simulink model "ISO_PID"  (R2018a)
settings: Solver=FixedStepAuto  StartTime=0.0  StopTime=3000  FixedStep=0.1  RelTol=1e-3
values from neighbouring files (symbols this model uses):
  f = [0,0]    [Model.m]
  h_T = [0 0]    [Model.m]
  hc = minreal(hc)    [Model.m]
libraries: simulink x2
settings Model: Creator=MinhKhanhPC  LastModifiedBy=thanhdo

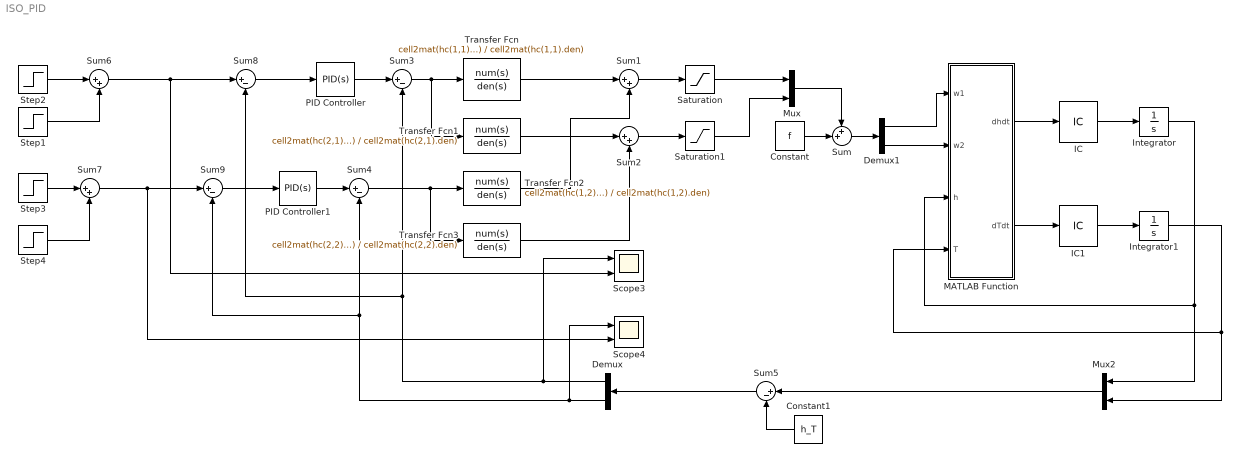
== system ISO_PID ==
  Constant : Constant  Value=f
  Constant1 : Constant  Value=h_T
  Demux : Demux  Outputs=2
  Demux1 : Demux  Outputs=2
  IC : InitialCondition  Value=0.1
  IC1 : InitialCondition  Value=30
  Integrator : Integrator  InitialCondition=0.1
  Integrator1 : Integrator  InitialCondition=30
  MATLAB Function : MATLAB Function  TreatAsAtomicUnit=on
  Mux : Mux  Inputs=2
  Mux2 : Mux  Inputs=2
  PID Controller : simulink/Continuous/PID Controller  Controller=PID  TimeDomain=Continuous-time  SampleTime=-1  IntegratorMethod=Forward Euler  FilterMethod=Forward Euler  Form=Parallel  UseFilter=on  ControllerParametersSource=internal  P=50  I=0.02  D=0  N=100  InitialConditionSource=internal  InitialConditionForIntegrator=0  InitialConditionForFilter=0  ExternalReset=none  LimitOutput=off  UpperSaturationLimit=inf  LowerSaturationLimit=-inf  LinearizeAsGain=on  AntiWindupMode=none  Kb=1  TrackingMode=off  Kt=1  PParamMin=[]  PParamMax=[]  IParamMin=[]  IParamMax=[]  DParamMin=[]  DParamMax=[]  NParamMin=[]  NParamMax=[]  KbParamMin=[]  KbParamMax=[]  KtParamMin=[]  KtParamMax=[]  POutMin=[]  POutMax=[]  IOutMin=[]  IOutMax=[]  DOutMin=[]  DOutMax=[]  NOutMin=[]  NOutMax=[]  KbOutMin=[]  KbOutMax=[]  KtOutMin=[]  KtOutMax=[]  IntegratorOutMin=[]  IntegratorOutMax=[]  FilterOutMin=[]  FilterOutMax=[]  SumOutMin=[]  SumOutMax=[]  SumI1OutMin=[]  SumI1OutMax=[]  SumI2OutMin=[]  SumI2OutMax=[]  SumI3OutMin=[]  SumI3OutMax=[]  SumDOutMin=[]  SumDOutMax=[]  SaturationOutMin=[]  SaturationOutMax=[]  IntegratorContinuousStateAttributes=''  IntegratorStateMustResolveToSignalObject=off  IntegratorRTWStateStorageClass=Auto  FilterContinuousStateAttributes=''  FilterStateMustResolveToSignalObject=off  FilterRTWStateStorageClass=Auto  DifferentiatorICPrevScaledInput=0  DifferentiatorOutMin=[]  DifferentiatorOutMax=[]  FilterDiffOutCoefMin=[]  FilterDiffOutCoefMax=[]  SumDenOutMin=[]  SumDenOutMax=[]  SumNumOutMin=[]  SumNumOutMax=[]  ReciprocalOutMin=[]  ReciprocalOutMax=[]  DivideOutMin=[]  DivideOutMax=[]  TunerSelectOption=Transfer Function Based (PID Tuner App)
  PID Controller1 : simulink/Continuous/PID Controller  Controller=PID  TimeDomain=Continuous-time  SampleTime=-1  IntegratorMethod=Forward Euler  FilterMethod=Forward Euler  Form=Parallel  UseFilter=on  ControllerParametersSource=internal  P=30  I=0  D=0  N=100  InitialConditionSource=internal  InitialConditionForIntegrator=0  InitialConditionForFilter=0  ExternalReset=none  LimitOutput=off  UpperSaturationLimit=inf  LowerSaturationLimit=-inf  LinearizeAsGain=on  AntiWindupMode=none  Kb=1  TrackingMode=off  Kt=1  PParamMin=[]  PParamMax=[]  IParamMin=[]  IParamMax=[]  DParamMin=[]  DParamMax=[]  NParamMin=[]  NParamMax=[]  KbParamMin=[]  KbParamMax=[]  KtParamMin=[]  KtParamMax=[]  POutMin=[]  POutMax=[]  IOutMin=[]  IOutMax=[]  DOutMin=[]  DOutMax=[]  NOutMin=[]  NOutMax=[]  KbOutMin=[]  KbOutMax=[]  KtOutMin=[]  KtOutMax=[]  IntegratorOutMin=[]  IntegratorOutMax=[]  FilterOutMin=[]  FilterOutMax=[]  SumOutMin=[]  SumOutMax=[]  SumI1OutMin=[]  SumI1OutMax=[]  SumI2OutMin=[]  SumI2OutMax=[]  SumI3OutMin=[]  SumI3OutMax=[]  SumDOutMin=[]  SumDOutMax=[]  SaturationOutMin=[]  SaturationOutMax=[]  IntegratorContinuousStateAttributes=''  IntegratorStateMustResolveToSignalObject=off  IntegratorRTWStateStorageClass=Auto  FilterContinuousStateAttributes=''  FilterStateMustResolveToSignalObject=off  FilterRTWStateStorageClass=Auto  DifferentiatorICPrevScaledInput=0  DifferentiatorOutMin=[]  DifferentiatorOutMax=[]  FilterDiffOutCoefMin=[]  FilterDiffOutCoefMax=[]  SumDenOutMin=[]  SumDenOutMax=[]  SumNumOutMin=[]  SumNumOutMax=[]  ReciprocalOutMin=[]  ReciprocalOutMax=[]  DivideOutMin=[]  DivideOutMax=[]  TunerSelectOption=Transfer Function Based (PID Tuner App)
  Saturation : Saturate  UpperLimit=4.28e-5  LowerLimit=0
  Saturation1 : Saturate  UpperLimit=2.28e-5  LowerLimit=0
  Scope3 : Scope  NumInputPorts=2
  Scope4 : Scope  NumInputPorts=2
  Step1 : Step  Time=1000  After=0.05  SampleTime=0
  Step2 : Step  After=0.05  SampleTime=0
  Step3 : Step  After=-5  SampleTime=0
  Step4 : Step  Time=2000  After=3  SampleTime=0
  Sum : Sum  Inputs=++|
  Sum{1..2,6..7} (4 alike) : Sum  Inputs=|++
  Sum{3..5,8..9} (5 alike) : Sum  Inputs=|+-
  Transfer Fcn : TransferFcn  Numerator=cell2mat(hc(1,1).num)  Denominator=cell2mat(hc(1,1).den)
  Transfer Fcn1 : TransferFcn  Numerator=cell2mat(hc(2,1).num)  Denominator=cell2mat(hc(2,1).den)
  Transfer Fcn2 : TransferFcn  Numerator=cell2mat(hc(1,2).num)  Denominator=cell2mat(hc(1,2).den)
  Transfer Fcn3 : TransferFcn  Numerator=cell2mat(hc(2,2).num)  Denominator=cell2mat(hc(2,2).den)
  wires:
  MATLAB Function/1(dhdt) -> IC/1
  Integrator/1 -> Mux2/1, MATLAB Function/3(h)
  Transfer Fcn3/1 -> Sum2/2
  Demux/2 -> Sum9/2, Sum4/2, Scope4/1
  Sum3/1 -> Transfer Fcn1/1, Transfer Fcn/1
  Demux/1 -> Sum8/2, Sum3/2, Scope3/1
  Transfer Fcn1/1 -> Sum2/1
  Transfer Fcn/1 -> Sum1/1
  Transfer Fcn2/1 -> Sum1/2
  Sum4/1 -> Transfer Fcn3/1, Transfer Fcn2/1
  Saturation/1 -> Mux/1
  Saturation1/1 -> Mux/2
  Sum5/1 -> Demux/1
  Constant1/1 -> Sum5/2
  Sum1/1 -> Saturation/1
  Sum2/1 -> Saturation1/1
  Sum/1 -> Demux1/1
  Demux1/1 -> MATLAB Function/1(w1)
  Demux1/2 -> MATLAB Function/2(w2)
  MATLAB Function/2(dTdt) -> IC1/1
  Integrator1/1 -> MATLAB Function/4(T), Mux2/2
  Mux2/1 -> Sum5/1
  IC/1 -> Integrator/1
  IC1/1 -> Integrator1/1
  Step2/1 -> Sum6/1
  Step1/1 -> Sum6/2
  Step3/1 -> Sum7/1
  Step4/1 -> Sum7/2
  PID Controller1/1 -> Sum4/1
  PID Controller/1 -> Sum3/1
  Sum8/1 -> PID Controller/1
  Sum9/1 -> PID Controller1/1
  Constant/1 -> Sum/2
  Mux/1 -> Sum/1
  Sum6/1 -> Scope3/2, Sum8/1
  Sum7/1 -> Scope4/2, Sum9/1

== matlab function ISO_PID/MATLAB Function ==
  data: w1 input; dhdt output; w2 input; h input; T input; dTdt output
function [dhdt, dTdt] = fcn(w1, w2, h, T)
%parameters
A = 3.24e-2; %area of tank
Th = 70;
Tc = 30;
g = 9.8;
%valve
Av = 7.85e-5;  %cross area 
v = 0.2;    %open-rate
% k = Av*sqrt(2*g) * v;
f3_max= 4.7e-5;
k= f3_max/sqrt(0.3);


dhdt = (w1 + w2 - k*sqrt(h))/A;
dTdt = (w1*(Tc - T) - w2*(T - Th))/(A*h);
